simulink model "LS_mag"  (R2016b)
settings: Solver=FixedStepAuto  StartTime=0.0  StopTime=5400  RelTol=1e-3
values from neighbouring files (symbols this model uses):
  TLE = fsw_params.bus.orbit_tle    [LS_mag_init.m]    (also in get_tle.m = tline2)
undefined symbols (not defined in the file or in its folder): GPS_time_lib, sim_params
libraries: mag_vec_lib x1, sgp4_lib_fsw x1, time_coord_rotation_lib x1
settings Model: Creator=Taylor  LastModifiedBy=Taylor

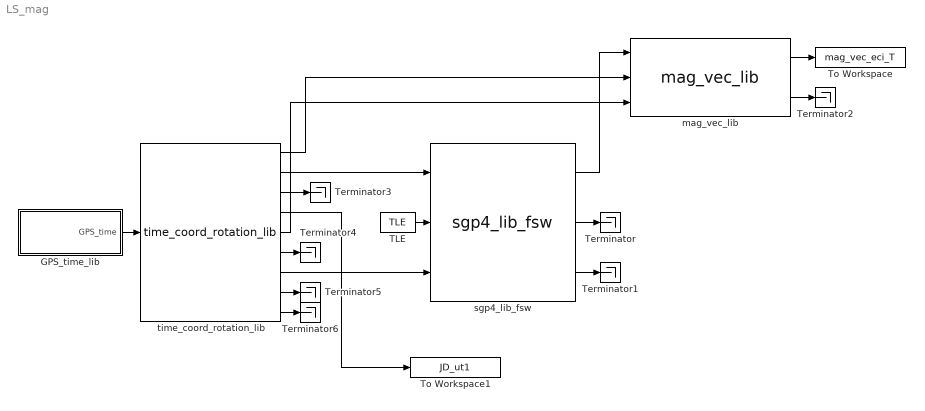
== system LS_mag ==
  GPS_time_lib : Subsystem  AncestorBlock=GPS_time_lib/GPS_time_lib
  TLE : Constant  Value=TLE
  Terminator{,1..6} (7 alike) : Terminator
  To Workspace : ToWorkspace  VariableName=mag_vec_eci_T  SampleTime=-1
  To Workspace1 : ToWorkspace  VariableName=JD_ut1  SampleTime=-1
  mag_vec_lib : mag_vec_lib/mag_vec_lib
  sgp4_lib_fsw : sgp4_lib_fsw/sgp4_lib_fsw
  time_coord_rotation_lib : time_coord_rotation_lib/time_coord_rotation_lib
  wires:
  GPS_time_lib/1(GPS_time) -> time_coord_rotation_lib/1
  time_coord_rotation_lib/5 -> mag_vec_lib/3
  time_coord_rotation_lib/1 -> mag_vec_lib/2
  sgp4_lib_fsw/1 -> mag_vec_lib/1
  sgp4_lib_fsw/2 -> Terminator/1
  sgp4_lib_fsw/3 -> Terminator1/1
  time_coord_rotation_lib/2 -> sgp4_lib_fsw/1
  time_coord_rotation_lib/7 -> sgp4_lib_fsw/3
  TLE/1 -> sgp4_lib_fsw/2
  time_coord_rotation_lib/3 -> Terminator3/1
  time_coord_rotation_lib/4 -> To Workspace1/1
  time_coord_rotation_lib/6 -> Terminator4/1
  time_coord_rotation_lib/8 -> Terminator5/1
  time_coord_rotation_lib/9 -> Terminator6/1
  mag_vec_lib/1 -> To Workspace/1
  mag_vec_lib/2 -> Terminator2/1

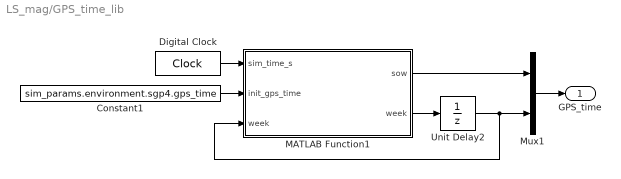
== system LS_mag/GPS_time_lib ==
  Constant1 : Constant  Value=sim_params.environment.sgp4.gps_time
  Digital Clock : DigitalClock  SampleTime=sim_params.sample_time_s
  MATLAB Function1 : MATLAB Function  TreatAsAtomicUnit=on
  Mux1 : Mux  Inputs=2
  Unit Delay2 : UnitDelay  InitialCondition=sim_params.environment.sgp4.gps_week_init  SampleTime=-1
  GPS_time : Outport
  wires:
  Mux1/1 -> GPS_time/1
  MATLAB Function1/1(sow) -> Mux1/1
  Unit Delay2/1 -> Mux1/2, MATLAB Function1/3("week ")
  MATLAB Function1/2(week) -> Unit Delay2/1
  Constant1/1 -> MATLAB Function1/2(init_gps_time)
  Digital Clock/1 -> MATLAB Function1/1(sim_time_s)

== matlab function LS_mag/GPS_time_lib/MATLAB Function1 ==
  data: sim_time_s input; sow output; init_gps_time input; week input; week output
function [sow, week] = gps_clock(sim_time_s, init_gps_time, week)
% ----------------------------------------------------------------------- %
% UW HuskySat-1, ADCS Subsystem
%
% GPS clock for the SIM.
% ----------------------------------------------------------------------- %

% Constants
sec_in_week = 604800;


init_sow    = init_gps_time(1);
sow         = mod(init_sow + sim_time_s, sec_in_week);

% Handle roll overs
if sow == sec_in_week
    week = week + 1;
end

end
